simulink model "Ejercicio1_09_03_17"  (R2013a)
settings: Solver=ode45  StartTime=0.0  StopTime=10.0  RelTol=1e-3
libraries: powerlib x10, powerlib_meascontrol x3
settings Model: Creator=Miguel  LastModifiedBy=Miguel

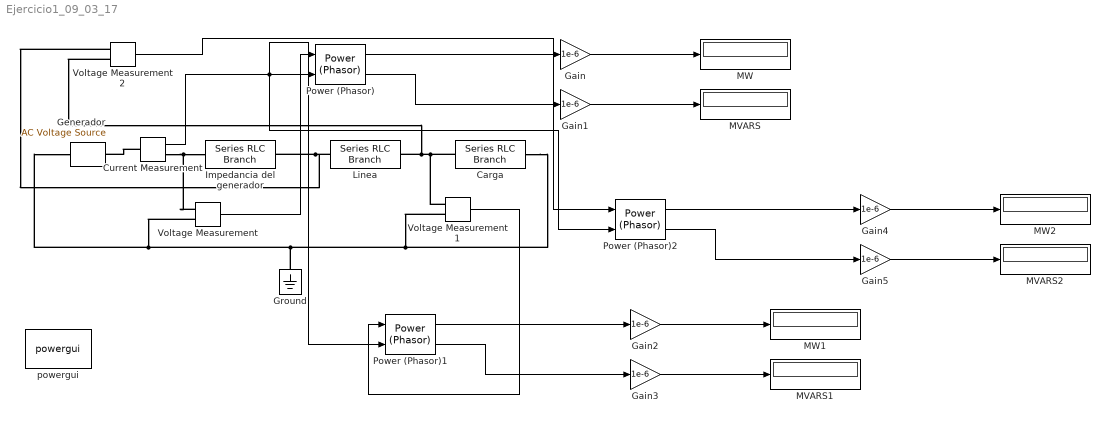
== system Ejercicio1_09_03_17 ==
  Carga : powerlib/Elements/Series RLC Branch  LConnTagsString=__new0  RConnTagsString=__new0  BranchType=RL  Resistance=65  Inductance=55/(2*pi*60)  SetiL0=off  InitialCurrent=0  Capacitance=1e-6  Setx0=off  InitialVoltage=0  Measurements=None
  Current Measurement : powerlib/Measurements/Current Measurement  PhasorSimulation=on  OutputType=Complex  PSBequivalent=0
  Gain{,1..5} (6 alike) : Gain  Gain=1e-6
  Generador : powerlib/Electrical Sources/AC Voltage Source  Amplitude=66.972e3*sqrt(2)  Phase=0  Frequency=60  SampleTime=0  Measurements=None
  Ground : powerlib/Elements/Ground  LConnTagsString=a
  Impedancia del generador : powerlib/Elements/Series RLC Branch  LConnTagsString=__new0  RConnTagsString=__new0  BranchType=L  Resistance=1  Inductance=10/(2*pi*60)  SetiL0=off  InitialCurrent=0  Capacitance=1e-6  Setx0=off  InitialVoltage=0  Measurements=None
  Linea : powerlib/Elements/Series RLC Branch  LConnTagsString=__new0  RConnTagsString=__new0  BranchType=RL  Resistance=1  Inductance=2/(2*pi*60)  SetiL0=off  InitialCurrent=0  Capacitance=1e-6  Setx0=off  InitialVoltage=0  Measurements=None
  MVARS : Display
  MVARS1 : Display
  MVARS2 : Display
  MW : Display
  MW1 : Display
  MW2 : Display
  Power (Phasor) : powerlib_meascontrol/Measurements/Power (Phasor)
  Power (Phasor)1 : powerlib_meascontrol/Measurements/Power (Phasor)
  Power (Phasor)2 : powerlib_meascontrol/Measurements/Power (Phasor)
  Voltage Measurement : powerlib/Measurements/Voltage Measurement  PhasorSimulation=on  OutputType=Complex  PSBequivalent=0
  Voltage Measurement1 : powerlib/Measurements/Voltage Measurement  PhasorSimulation=on  OutputType=Complex  PSBequivalent=0
  Voltage Measurement2 : powerlib/Measurements/Voltage Measurement  PhasorSimulation=on  OutputType=Complex  PSBequivalent=0
  powergui : powerlib/powergui  Priority=1  SimulationMode=Phasor  SolverType=Tustin  SampleTime=50e-6  frequency=60  SPID=off  DisableSnubberDevices=off  DisableRonSwitches=off  DisableVfSwitches=off  SwTol=0  Interpol=off  DisplayEquations=off  frequencyindice=60  Pbase=100e6  ErrMax=1e-4  Iterations=50  UnitsV=kV  UnitsW=MW  FunctionMessages=off  echomessages=off  HookPort=off  EnableUseOfTLC=off  x0status=blocks  RestoreLinks=warning  ResistiveCurrentMeasurement=off  Frange=[0:2:500]  Ylog=off  Xlog=on  ShowGrid=off  save=off  variable=ZData  ZoomFFT=off  StartTime=0.0  cycles=1  DisplayStyle=1  fundamental=60  FreqAxis=off  MaxFrequency=1000  frequencyindicesteady=1  RmsSteady=2  display=off  Ts=0  methode=off
  wires:
  Voltage Measurement/1 -> Power (Phasor)/1
  Power (Phasor)/1 -> Gain/1
  Power (Phasor)/2 -> Gain1/1
  Current Measurement/1 -> Power (Phasor)2/2, Power (Phasor)1/2, Power (Phasor)/2
  Gain/1 -> MW/1
  Gain1/1 -> MVARS/1
  Power (Phasor)1/1 -> Gain2/1
  Power (Phasor)1/2 -> Gain3/1
  Gain2/1 -> MW1/1
  Gain3/1 -> MVARS1/1
  Voltage Measurement1/1 -> Power (Phasor)1/1
  Power (Phasor)2/1 -> Gain4/1
  Power (Phasor)2/2 -> Gain5/1
  Gain4/1 -> MW2/1
  Gain5/1 -> MVARS2/1
  Voltage Measurement2/1 -> Power (Phasor)2/1
  connections:
  Linea/LConn1 -- Impedancia del generador/RConn1 -- Voltage Measurement2/LConn1
  Carga/LConn1 -- Voltage Measurement1/LConn1 -- Voltage Measurement2/LConn2 -- Linea/RConn1
  Carga/RConn1 -- Voltage Measurement1/LConn2 -- Ground/LConn1 -- Voltage Measurement/LConn2 -- Generador/LConn1
  Current Measurement/RConn1 -- Impedancia del generador/LConn1 -- Voltage Measurement/LConn1
  Current Measurement/LConn1 -- Generador/RConn1
